simulink model "DSB_SC"  (R2023a)
settings: Solver=VariableStepAuto  StartTime=0.0  StopTime=1  RelTol=1e-3
libraries: dspfdesign x1
settings Model: Creator=dung  LastModifiedBy=dung

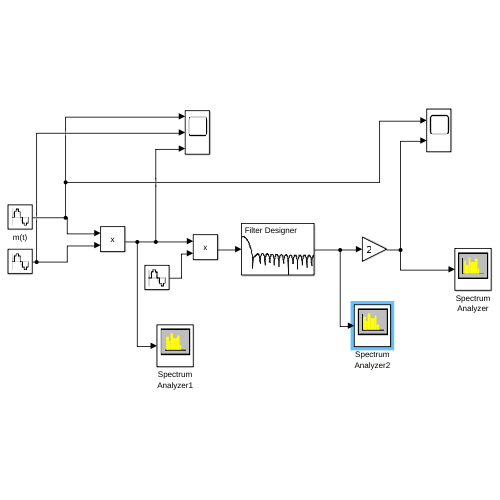
[thumbnail: Simulink's stored preview of the top-level diagram]
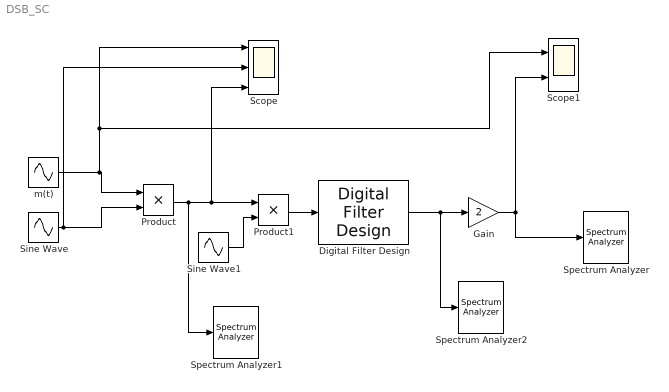
== system DSB_SC ==
  Digital Filter Design : dspfdesign/Digital Filter Design  mwdsp_browser_bugfix_var=off
  Gain : Gain  Gain=2
  Product : Product
  Product1 : Product
  Scope : Scope  NumInputPorts=3
  Scope1 : Scope  NumInputPorts=2
  Sine Wave : Sin  Frequency=2*pi*10000  SampleTime=1/100000
  Sine Wave1 : Sin  Frequency=2*pi*10000  SampleTime=1/100000
  Spectrum Analyzer : SpectrumAnalyzer  WindowPosition=[1.000000,265.000000,1397.000000,752.000000,]  ScopeFrameLocation=window  YLimits=[-225.06975346,50.94349227]  ColorLimits=[-20 80]  DefaultConfigurationName=spbscopes.SpectrumAnalyzerBlockCfg  IsFrequencyInputMode=0  FrequencyVectorPort=0  FrequencyVectorFromPort=0  FrequencyInputRBWPort=0  FrequencyInputRBWFromPort=0
  Spectrum Analyzer1 : SpectrumAnalyzer  WindowPosition=[560.000000,290.000000,800.000000,500.000000,]  ScopeFrameLocation=window  Span=99999.99999999999  StartFrequency=-49999.99999999999  StopFrequency=49999.99999999999  YLimits=[-210.2295906,43.31241752]  ColorLimits=[-20 80]  DefaultConfigurationName=spbscopes.SpectrumAnalyzerBlockCfg  IsFrequencyInputMode=0  FrequencyVectorPort=0  FrequencyVectorFromPort=0  FrequencyInputRBWPort=0  FrequencyInputRBWFromPort=0
  Spectrum Analyzer2 : SpectrumAnalyzer  WindowPosition=[560.000000,290.000000,800.000000,500.000000,]  ScopeFrameLocation=window  YLimits=[-84.99914459,28.65873844]  ColorLimits=[-20 80]  DefaultConfigurationName=spbscopes.SpectrumAnalyzerBlockCfg  IsFrequencyInputMode=0  FrequencyVectorPort=0  FrequencyVectorFromPort=0  FrequencyInputRBWPort=0  FrequencyInputRBWFromPort=0
  m(t) : Sin  Frequency=2*pi*1000  SampleTime=1/100000
  wires:
  m(t)/1 -> Scope1/1, Scope/1, Product/1
  Product/1 -> Spectrum Analyzer1/1, Product1/1, Scope/3
  Digital Filter Design/1 -> Spectrum Analyzer2/1, Gain/1
  Gain/1 -> Scope1/2, Spectrum Analyzer/1
  Product1/1 -> Digital Filter Design/1
  Sine Wave1/1 -> Product1/2
  Sine Wave/1 -> Scope/2, Product/2
